simulink model "simulacao"  (R2025a)
settings: Solver=VariableStepAuto  StartTime=0.0  StopTime=2  RelTol=1e-3
values from neighbouring files (symbols this model uses):
  C = 1e-6    (= 1e-06)    [parametros.m]
  L = 1e-3    (= 0.001)    [parametros.m]
  R = 1e3    (= 1000)    [parametros.m]
settings Model: Creator=luiza  LastModifiedBy=luiza

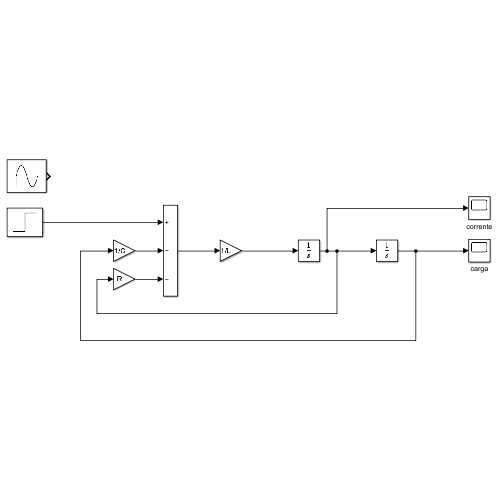
[thumbnail: Simulink's stored preview of the top-level diagram]
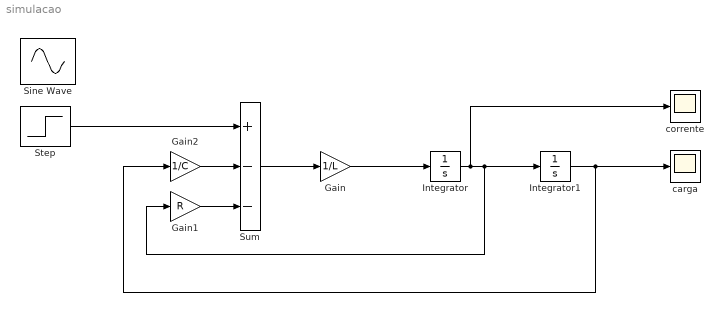
== system simulacao ==
  Gain : Gain  Gain=1/L
  Gain1 : Gain  Gain=R
  Gain2 : Gain  Gain=1/C
  Integrator : Integrator
  Integrator1 : Integrator
  Sine Wave : Sin  Amplitude=15  Frequency=20*pi  SampleTime=0
  Step : Step  Time=0  After=10  SampleTime=0
  Sum : Sum  Inputs=+--
  carga : Scope
      settings: ActiveDisplayYMinimum=-1.2500013000961666E-6  ActiveDisplayYMaximum=1.12500117008655E-5
  corrente : Scope
      settings: ActiveDisplayYMinimum=-0.0012539931077064864  ActiveDisplayYMaximum=0.011182034387814269
  wires:
  Sum/1 -> Gain/1
  Gain/1 -> Integrator/1
  Integrator/1 -> Integrator1/1, Gain1/1, corrente/1
  Integrator1/1 -> Gain2/1, carga/1
  Gain1/1 -> Sum/3
  Gain2/1 -> Sum/2
  Step/1 -> Sum/1
